simulink model "battery_cooling_ISO_2018cmpt"  (R2018b)
settings: Solver=FixedStepAuto  StartTime=0.0  StopTime=t_sim  FixedStep=1.0  MaxStep=1.0  RelTol=1e-2  AbsTol=1e-2
PreLoadFcn:
  | % Battery
  | battery.SOC_LUT = [0 0.1 0.25 0.5 0.75 0.9 1]';
  | battery.temperature_LUT = [5 20 40] + 273.15; %[K]
  | battery.capacity_LUT = [
  |     28.0081   27.6250   27.6392]; %[A*hr] Battery capacity
  | battery.Em_LUT = [
  |     3.4966    3.5057    3.5148
  |     3.5519    3.5660    3.5653
  |     3.6183    3.6337    3.6402
  |     3.7066    3.7127    3.7213
  |     3.9131    3.9259    3.9376
  |     4.0748    4.0777    4.0821
  |     4.1923    4.1928    4.1930]; % [Volts] Em open-circuit voltage vs SOC rows and T columns
  | battery.R0_LUT = [
  |     0.0117    0.0085    0.0090
  |     0.0110    0.0085    0.0090
  |     0.0114    0.0087    0.0092
  |     0.0107    0.0082    0.0088
  |     0.0107    0.0083    0.0091
  |     0.0113    0.0085    0.0089
  |     0.0116    0.0085    0.0089]; % [Ohms] R0 resistance vs SOC rows and T columns
  | battery.R1_LUT = [
  |     0.0109    0.0029    0.0013
  |     0.0069    0.0024    0.0012
  |     0.0047    0.0026    0.0013
  |     0.0034    0.0016    0.0010
  |     0.0033    0.0023    0.0014
  |     0.0033    0.0018    0.0011
  |     0.0028    0.0017    0.0011]; % [Ohms] R1 Resistance vs SOC rows and T columns
  | battery.C1_LUT = [
  |     1913.6    12447    30609
  |     4625.7    18872    32995
  |     23306     40764    47535
  |     10736     18721    26325
  |     18036     33630    48274
  |     12251     18360    26839
  |     9022.9    23394    30606]; % [Farads]  C1 Capacitance vs SOC rows and T columns
  | battery.cell_mass = 2.5; % [kg] Cell mass
  | battery.NCell = 20; % Number of cells per pack
  | battery.cell_Cp = 795; % [J/kg/K] Specific Heat
  | battery.Qe_init = 0; % [A*hr] Charge deficit
  | 
  | % Radiator
  | radiator.area_air = 0.15;                        % [m^2] Total cross sectional area (air)
  | radiator.volume_air = 0.01;                    % [m^3] Total volume (air)
  | radiator.area_liquid = pi*0.02^2/4;         % [m^2] Total cross sectional area (liquid)
  | radiator.volume_liquid = 2*pi*0.01^2/4;  % [m^3] Total volume (liquid)
  | radiator.mdot_air = [0.1  8];                   % [kg] Air mass flow rate
  | radiator.mdot_liquid = [0.1, 5];               % [kg] Liquid mass flow rate
  | radiator.SD = [ 1 9; 2 10];                      % [kW/K] Specific dissipation
  | radiator.dp_air = 1e-3*[3, 10];                % [MPa] Pressure drop (air)
  | radiator.dp_liquid = 1e-3*[5, 20];            % [MPa] Pressure drop (liquid)
  | 
  | % Pump
  | pump.omega = 4000;       % [RPM] Nominal angular velocity
  | pump.displacement = 40; % [cm^3/rev] Displacement
  | 
  | % Cooling channel
  | pipe.length = 75;                 % [cm] Length
  | pipe.Dh = 2.5;                     % [cm ] Hydraulic diameter
  | pipe.area = pi*pipe.Dh^2/4; % [cm^2] Cross sectional area
  | 
  | % 4-Way valve
  | valve.area = pipe.area;                % [cm^2] Cross sectional area
  | valve.opening = 0.98*valve.area;  % [cm^2] Maximum opening area
  | valve.area_leak = 1e-5;                % [cm^2] Leakage area
  | 
  | % Pressurized reservoir
  | tank.volume = 10;              % [l] Volume
  | tank.area = 0.25^2;           % [m^2] Cross-sectional area
  | tank.area_wall = 6*0.25^2; % [m^2] Wall surface area
  | 
  | T_set = 20.5;                  % [C] Batteries set point temperature
  | T_env =  30;                   % [C]  Outside temperature
  | T_init = T_env + 273.15;  % [K] Cooling liquid initial temperature
  | mdot_rev = 0.01;   %[kg/s] Reversal mass flow rate threshold
  | t_sim = 2474; % Simulation time
  | 
  | %pyenv(Version="/home/ananth/main/BTM/.venv/bin/python3.12", ExecutionMode="InProcess")
  | %setenv("ACADOS_SOURCE_DIR", "/home/ananth/main/BTM/acados")
libraries: SignalEditorBlockLib x1
CloseFcn:
  | try,close(h1_EVBatteryCoolingSystem),end
  | clear h1_EVBatteryCoolingSystem
  | try,close(h2_EVBatteryCoolingSystem),end
  | clear h2_EVBatteryCoolingSystem
  | try,close(h3_EVBatteryCoolingSystem),end
  | clear h3_EVBatteryCoolingSystem
  | try,close(h4_EVBatteryCoolingSystem),end
  | clear h4_EVBatteryCoolingSystem
  | 
  | clear SOC_LUT Temperature_LUT Capacity_LUT Em_LUT R0_LUT  R1_LUT
  | clear C1_LUT cell_mass NCell T_set T_env T_init radiator pump pipe valve
  | clear tank battery t_sim mdot_rev Qe_init
  | clear simlog_EVBatteryCoolingSystem tout
Description:
  | EV Battery Cooling System
settings Model: Tag=CustomStyle  Creator=The MathWorks, Inc.  LastModifiedBy=ananth
settings SolverCC: AutoScaleAbsTol=off  MaxConsecutiveMinStep=3  DecoupledContinuousIntegration=on  MinimalZcImpactIntegration=on
settings DataIOCC: MaxDataPoints=15000  SignalLoggingName=logsout_EVBatteryCoolingSystem
settings ConfigComp: CovBoundaryAbsTol=1.0e-5
settings SimscapeCC: SimscapeLogType=all  SimscapeLogSimulationStatistics=on  SimscapeLogName=simlog_EVBatteryCoolingSystem  SimscapeLogDataHistory=15000

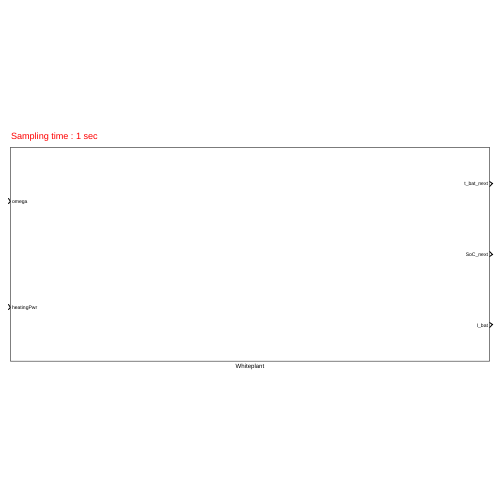
[thumbnail: Simulink's stored preview of the top-level diagram]
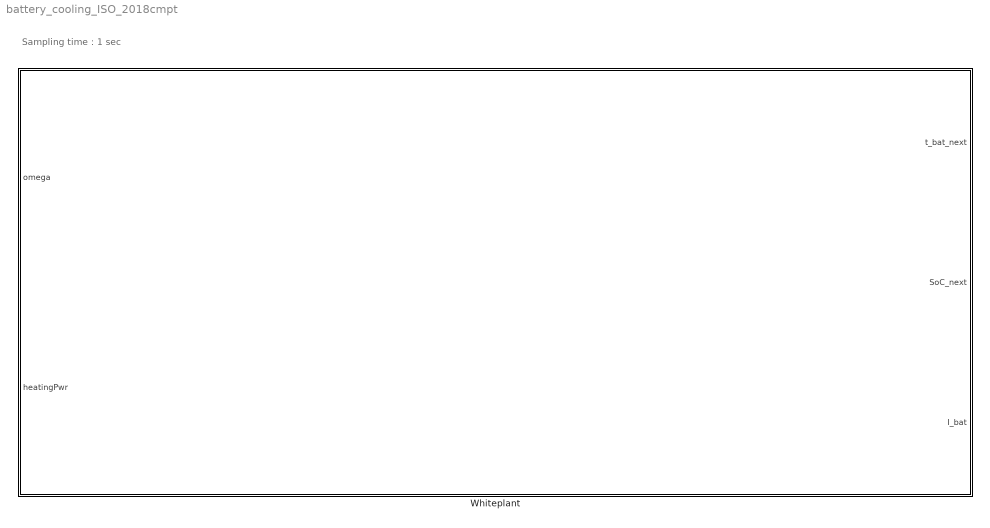
== system battery_cooling_ISO_2018cmpt ==
  note: Sampling time : 1 sec
  Whiteplant : Subsystem

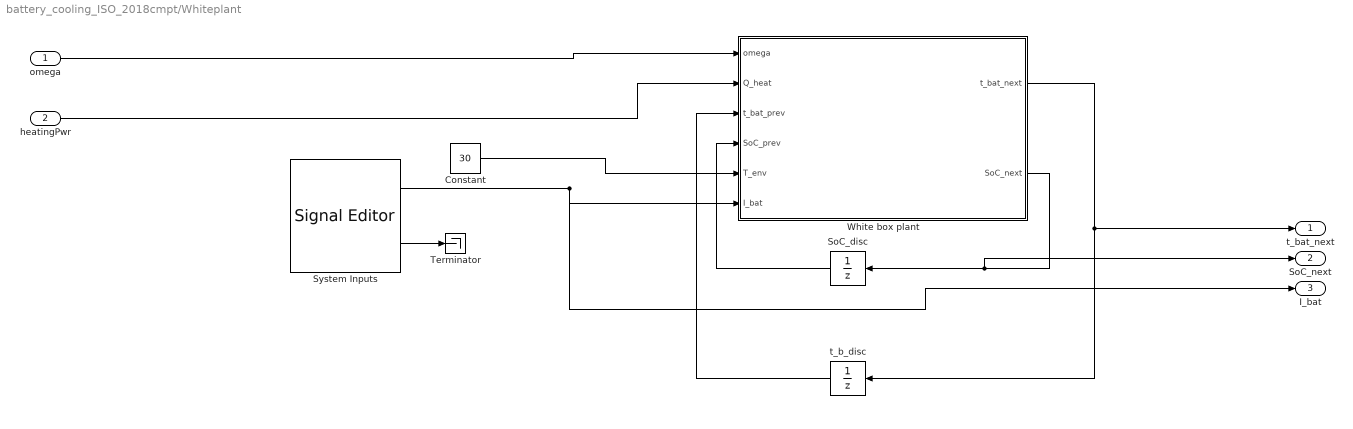
== system battery_cooling_ISO_2018cmpt/Whiteplant ==
  omega : Inport
  heatingPwr : Inport  Port=2
  Constant : Constant  Value=30
  SoC_disc : UnitDelay  InitialCondition=1  SampleTime=-1  HasFrameUpgradeWarning=on
  System Inputs : SignalEditorBlockLib/Signal Editor  FileName=EV_Extended.mat  ActiveScenario=FTP_75_Extended  ActiveSignal=current_ts  IsBus=off  OutputBusObjectStr=Bus: BusObject  SampleTime=0  Interpolate=off  ZeroCross=off  OutputAfterFinalValue=Setting to zero  Unit=inherit
  Terminator : Terminator
  White box plant : MATLAB Function  TreatAsAtomicUnit=on
  t_b_disc : UnitDelay  InitialCondition=30.0  SampleTime=-1  HasFrameUpgradeWarning=on
  t_bat_next : Outport
  SoC_next : Outport  Port=2
  I_bat : Outport  Port=3
  wires:
  SoC_disc/1 -> White box plant/4(SoC_prev)
  System Inputs/2 -> Terminator/1
  heatingPwr/1 -> White box plant/2(Q_heat)
  System Inputs/1 -> I_bat/1, White box plant/6(I_bat)
  t_b_disc/1 -> White box plant/3(t_bat_prev)
  Constant/1 -> White box plant/5(T_env)
  White box plant/1(t_bat_next) -> t_bat_next/1, t_b_disc/1
  omega/1 -> White box plant/1(omega)
  White box plant/2(SoC_next) -> SoC_next/1, SoC_disc/1

== matlab function battery_cooling_ISO_2018cmpt/Whiteplant/White box plant ==
  data: omega input; Q_heat input; t_bat_next output; t_bat_prev input; SoC_prev input; T_env input; I_bat input; SoC_next output
function [t_bat_next,SoC_next]  = whtbx(omega,Q_heat,t_bat_prev,SoC_prev,T_env,I_bat)

    % fixed params
    sample_time       = 1.0     ;
    alpha_0           = 0.635039;
    alpha_1           = 0.915692;
    alpha_2           = 0.919681;
    alpha_3           = 1.47275 ;
    gamma             = 7.38325 ;
    m_bat             = 20*2.5*4;
    c_bat             = 795     ;
    c_cool            = 3500    ;
    dens_cool         = 1050    ;
    pump_displacement = 1/(2*pi)*40/(100^3);
    R_bat             = 4*20*0.0128;
    C_bat             = 28*3600 ;
    h_A_bat           = 2500    ;


    % helper fucntions 
    m_dot_cool        = dens_cool*pump_displacement*omega;
    den               = m_dot_cool*c_cool + 1e-3;
    NTU_bat           = (alpha_3*h_A_bat)/den;
    t_cool_in         = t_bat_prev + alpha_1*(1/(1-exp(-NTU_bat)))*(Q_heat/den);
    t_cool_out        = (t_cool_in-t_bat_prev)*alpha_2*exp(-NTU_bat)+t_bat_prev;
    Q_cool            = m_dot_cool*c_cool*(t_cool_out-t_cool_in);



    % dynamics -> euler integration 
    t_bat_next        = t_bat_prev+(sample_time*(alpha_0/(m_bat*c_bat))*(I_bat^2*R_bat-Q_cool+gamma*(T_env-t_bat_prev)));
    SoC_next          = SoC_prev+(sample_time*(-I_bat/C_bat));
